simulink model "Learning_Example_run"  (R2020b)
settings: Solver=VariableStepAuto  StartTime=0.0  StopTime=50  RelTol=1e-3
values from neighbouring files (symbols this model uses):
  delta_time = 0.0178961433409    [Angular_gust.mat]    (also in Linear_gust.mat; Real_Values.m = time/length(xdata); Trial_Script.m = time/length(xdata); TryingNewAeroCoeffs.m = time/length(xdata))
  Fb1_l = -2600    [Angular_gust.mat]    (also in Linear_gust.mat; Real_Values.m = -260; Trial_Script.m; TryingNewAeroCoeffs.m)
  Fb1_u = 2600    [Angular_gust.mat]    (also in Linear_gust.mat; Real_Values.m = 260; Trial_Script.m; TryingNewAeroCoeffs.m)
  Fb2_l = -2600    [Angular_gust.mat]    (also in Linear_gust.mat; Real_Values.m = -260; Trial_Script.m; TryingNewAeroCoeffs.m)
  Fb2_u = 2600    [Angular_gust.mat]    (also in Linear_gust.mat; Real_Values.m = 260; Trial_Script.m; TryingNewAeroCoeffs.m)
  Fb3_l = -3200    [Angular_gust.mat]    (also in Linear_gust.mat; Real_Values.m = -320; Trial_Script.m; TryingNewAeroCoeffs.m)
  Fb3_u = 3200    [Angular_gust.mat]    (also in Linear_gust.mat; Real_Values.m = 320; Trial_Script.m; TryingNewAeroCoeffs.m)
  Fb4_l = -3200    [Angular_gust.mat]    (also in Linear_gust.mat; Real_Values.m = -320; Trial_Script.m; TryingNewAeroCoeffs.m)
  Fb4_u = 3200    [Angular_gust.mat]    (also in Linear_gust.mat; Real_Values.m = 320; Trial_Script.m; TryingNewAeroCoeffs.m)
  Fc1_l = -300    [Angular_gust.mat]    (also in Linear_gust.mat; Real_Values.m = -100; Trial_Script.m = -3000; TryingNewAeroCoeffs.m)
  Fc1_u = 300    [Angular_gust.mat]    (also in Linear_gust.mat; Real_Values.m = 100; Trial_Script.m = 3000; TryingNewAeroCoeffs.m)
  Fc2_l = -300    [Angular_gust.mat]    (also in Linear_gust.mat; Real_Values.m = -100; Trial_Script.m = -3000; TryingNewAeroCoeffs.m)
  Fc2_u = 300    [Angular_gust.mat]    (also in Linear_gust.mat; Real_Values.m = 100; Trial_Script.m = 3000; TryingNewAeroCoeffs.m)
  Fc3_l = -300    [Angular_gust.mat]    (also in Linear_gust.mat; Real_Values.m = -100; Trial_Script.m = -3000; TryingNewAeroCoeffs.m)
  Fc3_u = 300    [Angular_gust.mat]    (also in Linear_gust.mat; Real_Values.m = 100; Trial_Script.m = 3000; TryingNewAeroCoeffs.m)
  fprop = 1000    [Angular_gust.mat]    (also in Linear_gust.mat; TryingNewAeroCoeffs.m)
  Ft1_l = -5600    [Angular_gust.mat]    (also in Linear_gust.mat; Real_Values.m = -560; Trial_Script.m; TryingNewAeroCoeffs.m)
  Ft1_u = 5600    [Angular_gust.mat]    (also in Linear_gust.mat; Real_Values.m = 560; Trial_Script.m; TryingNewAeroCoeffs.m)
  Ft2_l = -5600    [Angular_gust.mat]    (also in Linear_gust.mat; Real_Values.m = -560; Trial_Script.m; TryingNewAeroCoeffs.m)
  Ft2_u = 5600    [Angular_gust.mat]    (also in Linear_gust.mat; Real_Values.m = 560; Trial_Script.m; TryingNewAeroCoeffs.m)
  Ft3_l = -3200    [Angular_gust.mat]    (also in Linear_gust.mat; Real_Values.m = -320; Trial_Script.m; TryingNewAeroCoeffs.m)
  Ft3_u = 3200    [Angular_gust.mat]    (also in Linear_gust.mat; Real_Values.m = 320; Trial_Script.m; TryingNewAeroCoeffs.m)
  Ft4_l = -3200    [Angular_gust.mat]    (also in Linear_gust.mat; Real_Values.m = -320; Trial_Script.m; TryingNewAeroCoeffs.m)
  Ft4_u = 3200    [Angular_gust.mat]    (also in Linear_gust.mat; Real_Values.m = 320; Trial_Script.m; TryingNewAeroCoeffs.m)
  g = 9.81    [Angular_gust.mat]    (also in Linear_gust.mat; Real_Values.m; Trial_Script.m; TryingNewAeroCoeffs.m)
  m = 941.102    [Angular_gust.mat]    (also in Linear_gust.mat; Real_Values.m; Trial_Script.m = 645; TryingNewAeroCoeffs.m)
  r_cgCatia = [0.0401998 0.00180957 -0.293434]    [Angular_gust.mat]    (also in Linear_gust.mat; Real_Values.m = TcgCatia*r_cgCatia; Trial_Script.m = [2; 0; 0]; TryingNewAeroCoeffs.m = TcgCatia*r_cgCatia)
  r_trajectory = [0 0 0]    [Angular_gust.mat]    (also in Linear_gust.mat; Real_Values.m = [0;0;0]; Trial_Script.m = [0;0;0]; TryingNewAeroCoeffs.m = [0;0;0])
  rho = 1.225    [Angular_gust.mat]    (also in Linear_gust.mat; Real_Values.m; Trial_Script.m; TryingNewAeroCoeffs.m)
  t_finalgust = 17.9140394843    [Angular_gust.mat]    (also in Linear_gust.mat; Real_Values.m = time; TryingNewAeroCoeffs.m = time)
  TcgCatia = [1  0  0; 0  -1  0; 0  0  -1]    [Angular_gust.mat]    (also in Linear_gust.mat; Real_Values.m = [1 0 0; Trial_Script.m = [1 0 0; TryingNewAeroCoeffs.m = [1 0 0)
  time = 17.9140394843    [Angular_gust.mat]    (also in Linear_gust.mat; Real_Values.m = rdiff_abs/V0_shard; Trial_Script.m = abs(rdiff_shard(2)/V0_shard(2)); TryingNewAeroCoeffs.m = rdiff_abs/V0_shard)
  time_delay = 0.01    [Angular_gust.mat]    (also in Linear_gust.mat; Real_Values.m = 0.1; Trial_Script.m = 0.1; TryingNewAeroCoeffs.m)
  Tzy_Shard = [6.12323399574e-17  1  1.22464679915e-16; 1  -6.12323399574e-17  -7.49879891331e-33; 0  1.22464679915e-16  -1]    [Angular_gust.mat]    (also in Linear_gust.mat; Real_Values.m = [cos(pi/2) -sin(pi/2) 0; sin(pi/2) cos(pi/2) 0; 0 0 1]*[1 0 ; Trial_Script.m = [cos(pi/2) -sin(pi/2) 0; sin(pi/2) cos(pi/2) 0; 0 0 1]*[1 0 ; TryingNewAeroCoeffs.m = [cos(pi/2) -sin(pi/2) 0; sin(pi/2) cos(pi/2) 0; 0 0 1]*[1 0 )
  u0_final = 23.9559    [Angular_gust.mat]    (also in Linear_gust.mat; Real_Values.m = u_0(length(u_0)); TryingNewAeroCoeffs.m = u_0(length(u_0)))
  u0_ini = 24.7775    [Angular_gust.mat]    (also in Linear_gust.mat; TryingNewAeroCoeffs.m = u_0(1))
  u1_final = -0.480858    [Angular_gust.mat]    (also in Linear_gust.mat; Real_Values.m = u_1(length(u_1)); TryingNewAeroCoeffs.m = u_1(length(u_1)))
  u1_ini = 0.712897    [Angular_gust.mat]    (also in Linear_gust.mat; TryingNewAeroCoeffs.m = u_1(1))
  u2_final = -0.725589    [Angular_gust.mat]    (also in Linear_gust.mat; Real_Values.m = u_2(length(u_2)); TryingNewAeroCoeffs.m = u_2(length(u_2)))
  u2_ini = -0.504815    [Angular_gust.mat]    (also in Linear_gust.mat; TryingNewAeroCoeffs.m = u_2(1))
  u_0 = [24.7775 24.7775 24.7775 24.7775 24.7775 24.7775 24.7775 24.7775 24.7775 24.7775 24.7775 24.7775 ... (1001 elements, 1001x1)]    [Angular_gust.mat]    (also in Linear_gust.mat; Real_Values.m = a(1:d_shard,1); Trial_Script.m = a(1:d_shard,1); TryingNewAeroCoeffs.m = a(1:d_shard,1))
  u_1 = [0.712897 0.712897 0.712897 0.712897 0.712897 0.712897 0.712897 0.712897 0.712897 0.712897 0.712897 0.712897 ... (1001 elements, 1001x1)]    [Angular_gust.mat]    (also in Linear_gust.mat; Real_Values.m = a(1:d_shard,2); Trial_Script.m = a(1:d_shard,2); TryingNewAeroCoeffs.m = a(1:d_shard,2))
  u_2 = [-0.504815 -0.504815 -0.504815 -0.504815 -0.504815 -0.504815 -0.504815 -0.504815 -0.504815 -0.504815 -0.504815 -0.504815 ... (1001 elements, 1001x1)]    [Angular_gust.mat]    (also in Linear_gust.mat; Real_Values.m = a(1:d_shard,3); Trial_Script.m = a(1:d_shard,3); TryingNewAeroCoeffs.m = a(1:d_shard,3))
  v_sh = [9.97862823256 -6.11014756245e-16 -13.3493354282]    [Angular_gust.mat]    (also in Linear_gust.mat; TryingNewAeroCoeffs.m = Tzy_Shard*[0; Vz0_shard; Vy0_shard])
  vq1 = interp1(out.tout,Fx_pre,xq)    [Learning_Code.m]    (also in PlottingSigmoidLeftover.m)
  vq2 = interp1(out.tout,Fy_pre,xq)    [Learning_Code.m]    (also in PlottingSigmoidLeftover.m)
  vq3 = interp1(out.tout,Fz_pre,xq)    [Learning_Code.m]    (also in PlottingSigmoidLeftover.m)
  xq = 0:0.001:40    [Learning_Code.m]    (also in PlottingSigmoidLeftover.m)
  ZI_Cx = [4.10002314469 4.10486511138 4.10970707807 4.11454904475 4.11939101144 4.12423297813 4.12907494481 4.1339169115 4.13875887819 4.14360084487 4.14844281156 4.15328477825 ... (65341 elements, 361x181)]    [Angular_gust.mat]    (also in Linear_gust.mat; Real_Values.m = model_Cx(XI_Cx, YI_Cx); Trial_Script.m = model_Cx(XI_Cx, YI_Cx); TryingNewAeroCoeffs.m = model_Cx(XI_Cx, YI_Cx))
  ZI_Cy = [5.10662222372 5.15407485934 5.20152749496 5.24898013059 5.29643276621 5.34388540184 5.39133803746 5.43879067308 5.48624330871 5.53369594433 5.58114857996 5.62860121558 ... (65341 elements, 361x181)]    [Angular_gust.mat]    (also in Linear_gust.mat; Real_Values.m = model_Cy(XI_Cy, YI_Cy); Trial_Script.m = model_Cy(XI_Cy, YI_Cy); TryingNewAeroCoeffs.m = model_Cy(XI_Cy, YI_Cy))
  ZI_Cz = [-10.5947720774 -10.6317912004 -10.6688103235 -10.7058294465 -10.7428485695 -10.7798676926 -10.8168868156 -10.8539059387 -10.8909250617 -10.9279441847 -10.9649633078 -11.0019824308 ... (65341 elements, 361x181)]    [Angular_gust.mat]    (also in Linear_gust.mat; Real_Values.m = model_Cz(XI_Cz, YI_Cz); Trial_Script.m = model_Cz(XI_Cz, YI_Cz); TryingNewAeroCoeffs.m = model_Cz(XI_Cz, YI_Cz))
  ZI_p = [6.05111971338 6.06712776392 6.08313581446 6.099143865 6.11515191553 6.13115996607 6.14716801661 6.16317606715 6.17918411769 6.19519216823 6.21120021877 6.22720826931 ... (65341 elements, 361x181)]    [Angular_gust.mat]    (also in Linear_gust.mat; Real_Values.m = model_p(XI_p, YI_p); Trial_Script.m = model_p(XI_p, YI_p); TryingNewAeroCoeffs.m = model_p(XI_p, YI_p))
  ZI_q = [0.071083987219 0.054175962948 0.0372679386771 0.0203599144061 0.00345189013513 -0.0134561341358 -0.0303641584068 -0.0472721826778 -0.0641802069487 -0.0810882312197 -0.0979962554907 -0.114904279762 ... (65341 elements, 361x181)]    [Angular_gust.mat]    (also in Linear_gust.mat; Real_Values.m = model_q(XI_q, YI_q); Trial_Script.m = model_q(XI_q, YI_q); TryingNewAeroCoeffs.m = model_q(XI_q, YI_q))
  ZI_r = [-1.8762921931 -1.88364224017 -1.89099228723 -1.8983423343 -1.90569238136 -1.91304242842 -1.92039247549 -1.92774252255 -1.93509256961 -1.94244261668 -1.94979266374 -1.95714271081 ... (65341 elements, 361x181)]    [Angular_gust.mat]    (also in Linear_gust.mat; Real_Values.m = model_r(XI_r, YI_r); Trial_Script.m = model_r(XI_r, YI_r); TryingNewAeroCoeffs.m = model_r(XI_r, YI_r))
libraries: dspsigops x11, simulink x6, pid_lib x3, sharedutil x1
settings Model: Creator=Jonathan van Zyl  LastModifiedBy=Jonathan van Zyl

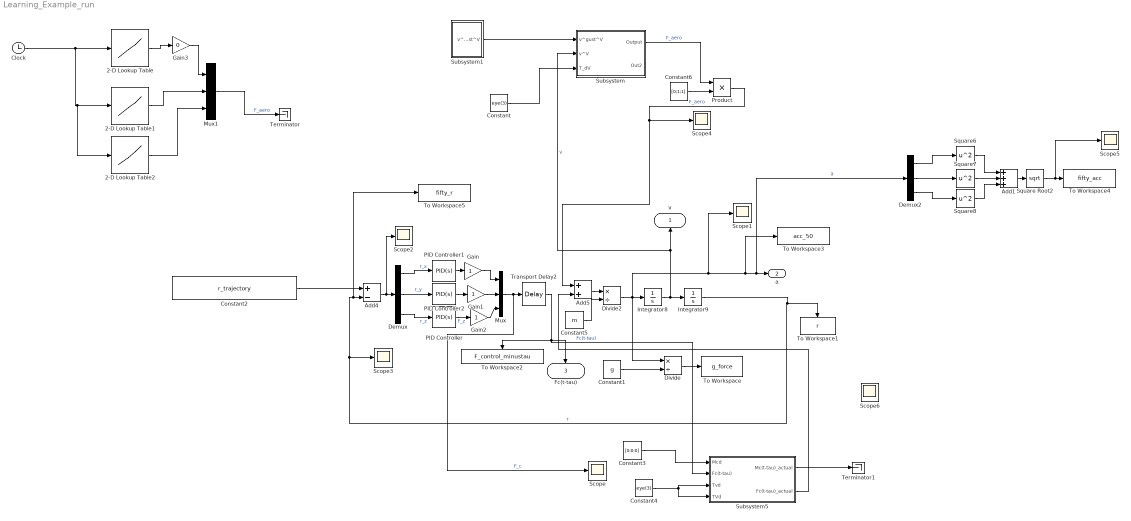
== system Learning_Example_run ==
  2-D Lookup Table : Lookup_n-D  NumberOfTableDimensions=1  BreakpointsForDimension1=xq  BreakpointsForDimension2=[0:1:40001]  Table=vq1  InternalRulePriority=Speed  RndMeth=Simplest  InputSameDT=on
  2-D Lookup Table1 : Lookup_n-D  NumberOfTableDimensions=1  BreakpointsForDimension1=xq  BreakpointsForDimension2=[0:1:40001]  Table=vq2  InternalRulePriority=Speed  RndMeth=Simplest  InputSameDT=on
  2-D Lookup Table2 : Lookup_n-D  NumberOfTableDimensions=1  BreakpointsForDimension1=xq  BreakpointsForDimension2=[0:1:40001]  Table=vq3  InternalRulePriority=Speed  RndMeth=Simplest  InputSameDT=on
  Add1 : Sum  Inputs=+++
  Add4 : Sum  Inputs=+-
  Add5 : Sum
  Clock : Clock
  Constant : Constant  Value=eye(3)
  Constant1 : Constant  Value=g
  Constant2 : Constant  Value=r_trajectory
  Constant3 : Constant  Value=[0;0;0]
  Constant4 : Constant  Value=eye(3)
  Constant5 : Constant  Value=m
  Constant6 : Constant  Value=[0;1;1]
  Demux : Demux  Outputs=3
  Demux2 : Demux  Outputs=3
  Divide : Product  Inputs=*/
  Divide2 : Product  Inputs=*/
  Gain : Gain
  Gain1 : Gain
  Gain2 : Gain
  Gain3 : Gain  Gain=0
  Integrator8 : Integrator
  Integrator9 : Integrator
  Mux : Mux  Inputs=3
  Mux1 : Mux  Inputs=3
  PID Controller : pid_lib/PID Controller  Controller=PID  Form=Parallel  TimeDomain=Continuous-time  UseExternalTs=off  SampleTime=-1  IntegratorMethod=Forward Euler  FilterMethod=Forward Euler  ControllerParametersSource=internal  P=165.49617069696  I=7.27585376172433  D=919.065111272192  UseFilter=on  N=5.45397025421619  TunerSelectOption=Transfer Function Based (PID Tuner App)  InitialConditionSource=internal  InitialConditionForIntegrator=0  InitialConditionForFilter=0  DifferentiatorICPrevScaledInput=0  ExternalReset=none  TrackingMode=off  Kt=1  LimitOutput=off  SatLimitsSource=internal  UpperSaturationLimit=inf  LowerSaturationLimit=-inf  LinearizeAsGain=on  AntiWindupMode=none  Kb=1  POutMin=[]  POutMax=[]  IOutMin=[]  IOutMax=[]  DOutMin=[]  DOutMax=[]  NOutMin=[]  NOutMax=[]  SumOutMin=[]  SumOutMax=[]  SaturationOutMin=[]  SaturationOutMax=[]  PParamMin=[]  PParamMax=[]  IParamMin=[]  IParamMax=[]  DParamMin=[]  DParamMax=[]  NParamMin=[]  NParamMax=[]  KbParamMin=[]  KbParamMax=[]  KtParamMin=[]  KtParamMax=[]  KbOutMin=[]  KbOutMax=[]  KtOutMin=[]  KtOutMax=[]  IntegratorOutMin=[]  IntegratorOutMax=[]  FilterOutMin=[]  FilterOutMax=[]  SumI1OutMin=[]  SumI1OutMax=[]  SumI2OutMin=[]  SumI2OutMax=[]  SumI3OutMin=[]  SumI3OutMax=[]  SumI4OutMin=[]  SumI4OutMax=[]  SumDOutMin=[]  SumDOutMax=[]  DifferentiatorOutMin=[]  DifferentiatorOutMax=[]  FilterDiffOutCoefMin=[]  FilterDiffOutCoefMax=[]  ReciprocalOutMin=[]  ReciprocalOutMax=[]  SumDenOutMin=[]  SumDenOutMax=[]  SumNumOutMin=[]  SumNumOutMax=[]  DivideOutMin=[]  DivideOutMax=[]  UdiffTsProdOutMin=[]  UdiffTsProdOutMax=[]  NTsProdOutMin=[]  NTsProdOutMax=[]  UintegralTsProdOutMin=[]  UintegralTsProdOutMax=[]  UngainTsProdOutMin=[]  UngainTsProdOutMax=[]  IntegratorContinuousStateAttributes=''  IntegratorStateMustResolveToSignalObject=off  IntegratorRTWStateStorageClass=Auto  FilterContinuousStateAttributes=''  FilterStateMustResolveToSignalObject=off  FilterRTWStateStorageClass=Auto  ParallelPVariant=InternalParameters  IdealPVariant=Disabled  IVariant=InternalParameters  DVariant=InternalParameters  IntegratorVariant=Continuous  SatVariant=Disabled  AWVariant=Passthrough  PCopyVariant=Disabled  TRVariant=Disabled  FdbkBlocksVariant=Forward  IdealPFdbkVariant=Disabled  SatFdbkVariant=Disabled  DerivativeFilterVariant=ContFilter  NVariant=InternalParameters  NCopyVariant=Disabled  FilterICVariant=InternalICsFilter  IntegratorICVariant=InternalICs  ExternalResetVariant=Disabled  TRSumVariant=Passthrough  SumFdbkVariant=Disabled  SumVariant=Sum_PID  TsampFilterVariant=InternalTs  TsampNgainVariant=Passthrough  TsampIntegralVariant=Passthrough  ExternalSaturationOutDataTypeStr=Inherit: Same as second input
  PID Controller1 : pid_lib/PID Controller  Controller=PID  Form=Parallel  TimeDomain=Continuous-time  UseExternalTs=off  SampleTime=-1  IntegratorMethod=Forward Euler  FilterMethod=Forward Euler  ControllerParametersSource=internal  P=118.225343121314  I=1.50893910785693  D=2058.11872086996  UseFilter=on  N=250.023518875976  TunerSelectOption=Transfer Function Based (PID Tuner App)  InitialConditionSource=internal  InitialConditionForIntegrator=0  InitialConditionForFilter=0  DifferentiatorICPrevScaledInput=0  ExternalReset=none  TrackingMode=off  Kt=1  LimitOutput=off  SatLimitsSource=internal  UpperSaturationLimit=inf  LowerSaturationLimit=-inf  LinearizeAsGain=on  AntiWindupMode=none  Kb=1  POutMin=[]  POutMax=[]  IOutMin=[]  IOutMax=[]  DOutMin=[]  DOutMax=[]  NOutMin=[]  NOutMax=[]  SumOutMin=[]  SumOutMax=[]  SaturationOutMin=[]  SaturationOutMax=[]  PParamMin=[]  PParamMax=[]  IParamMin=[]  IParamMax=[]  DParamMin=[]  DParamMax=[]  NParamMin=[]  NParamMax=[]  KbParamMin=[]  KbParamMax=[]  KtParamMin=[]  KtParamMax=[]  KbOutMin=[]  KbOutMax=[]  KtOutMin=[]  KtOutMax=[]  IntegratorOutMin=[]  IntegratorOutMax=[]  FilterOutMin=[]  FilterOutMax=[]  SumI1OutMin=[]  SumI1OutMax=[]  SumI2OutMin=[]  SumI2OutMax=[]  SumI3OutMin=[]  SumI3OutMax=[]  SumI4OutMin=[]  SumI4OutMax=[]  SumDOutMin=[]  SumDOutMax=[]  DifferentiatorOutMin=[]  DifferentiatorOutMax=[]  FilterDiffOutCoefMin=[]  FilterDiffOutCoefMax=[]  ReciprocalOutMin=[]  ReciprocalOutMax=[]  SumDenOutMin=[]  SumDenOutMax=[]  SumNumOutMin=[]  SumNumOutMax=[]  DivideOutMin=[]  DivideOutMax=[]  UdiffTsProdOutMin=[]  UdiffTsProdOutMax=[]  NTsProdOutMin=[]  NTsProdOutMax=[]  UintegralTsProdOutMin=[]  UintegralTsProdOutMax=[]  UngainTsProdOutMin=[]  UngainTsProdOutMax=[]  IntegratorContinuousStateAttributes=''  IntegratorStateMustResolveToSignalObject=off  IntegratorRTWStateStorageClass=Auto  FilterContinuousStateAttributes=''  FilterStateMustResolveToSignalObject=off  FilterRTWStateStorageClass=Auto  ParallelPVariant=InternalParameters  IdealPVariant=Disabled  IVariant=InternalParameters  DVariant=InternalParameters  IntegratorVariant=Continuous  SatVariant=Disabled  AWVariant=Passthrough  PCopyVariant=Disabled  TRVariant=Disabled  FdbkBlocksVariant=Forward  IdealPFdbkVariant=Disabled  SatFdbkVariant=Disabled  DerivativeFilterVariant=ContFilter  NVariant=InternalParameters  NCopyVariant=Disabled  FilterICVariant=InternalICsFilter  IntegratorICVariant=InternalICs  ExternalResetVariant=Disabled  TRSumVariant=Passthrough  SumFdbkVariant=Disabled  SumVariant=Sum_PID  TsampFilterVariant=InternalTs  TsampNgainVariant=Passthrough  TsampIntegralVariant=Passthrough  ExternalSaturationOutDataTypeStr=Inherit: Same as second input
  PID Controller2 : pid_lib/PID Controller  Controller=PID  Form=Parallel  TimeDomain=Continuous-time  UseExternalTs=off  SampleTime=-1  IntegratorMethod=Forward Euler  FilterMethod=Forward Euler  ControllerParametersSource=internal  P=165.49617069696  I=7.27585376172433  D=919.065111272192  UseFilter=on  N=5.45397025421619  TunerSelectOption=Transfer Function Based (PID Tuner App)  InitialConditionSource=internal  InitialConditionForIntegrator=0  InitialConditionForFilter=0  DifferentiatorICPrevScaledInput=0  ExternalReset=none  TrackingMode=off  Kt=1  LimitOutput=off  SatLimitsSource=internal  UpperSaturationLimit=inf  LowerSaturationLimit=-inf  LinearizeAsGain=on  AntiWindupMode=none  Kb=1  POutMin=[]  POutMax=[]  IOutMin=[]  IOutMax=[]  DOutMin=[]  DOutMax=[]  NOutMin=[]  NOutMax=[]  SumOutMin=[]  SumOutMax=[]  SaturationOutMin=[]  SaturationOutMax=[]  PParamMin=[]  PParamMax=[]  IParamMin=[]  IParamMax=[]  DParamMin=[]  DParamMax=[]  NParamMin=[]  NParamMax=[]  KbParamMin=[]  KbParamMax=[]  KtParamMin=[]  KtParamMax=[]  KbOutMin=[]  KbOutMax=[]  KtOutMin=[]  KtOutMax=[]  IntegratorOutMin=[]  IntegratorOutMax=[]  FilterOutMin=[]  FilterOutMax=[]  SumI1OutMin=[]  SumI1OutMax=[]  SumI2OutMin=[]  SumI2OutMax=[]  SumI3OutMin=[]  SumI3OutMax=[]  SumI4OutMin=[]  SumI4OutMax=[]  SumDOutMin=[]  SumDOutMax=[]  DifferentiatorOutMin=[]  DifferentiatorOutMax=[]  FilterDiffOutCoefMin=[]  FilterDiffOutCoefMax=[]  ReciprocalOutMin=[]  ReciprocalOutMax=[]  SumDenOutMin=[]  SumDenOutMax=[]  SumNumOutMin=[]  SumNumOutMax=[]  DivideOutMin=[]  DivideOutMax=[]  UdiffTsProdOutMin=[]  UdiffTsProdOutMax=[]  NTsProdOutMin=[]  NTsProdOutMax=[]  UintegralTsProdOutMin=[]  UintegralTsProdOutMax=[]  UngainTsProdOutMin=[]  UngainTsProdOutMax=[]  IntegratorContinuousStateAttributes=''  IntegratorStateMustResolveToSignalObject=off  IntegratorRTWStateStorageClass=Auto  FilterContinuousStateAttributes=''  FilterStateMustResolveToSignalObject=off  FilterRTWStateStorageClass=Auto  ParallelPVariant=InternalParameters  IdealPVariant=Disabled  IVariant=InternalParameters  DVariant=InternalParameters  IntegratorVariant=Continuous  SatVariant=Disabled  AWVariant=Passthrough  PCopyVariant=Disabled  TRVariant=Disabled  FdbkBlocksVariant=Forward  IdealPFdbkVariant=Disabled  SatFdbkVariant=Disabled  DerivativeFilterVariant=ContFilter  NVariant=InternalParameters  NCopyVariant=Disabled  FilterICVariant=InternalICsFilter  IntegratorICVariant=InternalICs  ExternalResetVariant=Disabled  TRSumVariant=Passthrough  SumFdbkVariant=Disabled  SumVariant=Sum_PID  TsampFilterVariant=InternalTs  TsampNgainVariant=Passthrough  TsampIntegralVariant=Passthrough  ExternalSaturationOutDataTypeStr=Inherit: Same as second input
  Product : Product
  Scope{,1..6} (7 alike) : Scope
  Square Root2 : Sqrt  SaturateOnIntegerOverflow=on
  Square6 : Math  Operator=square  SaturateOnIntegerOverflow=on
  Square7 : Math  Operator=square  SaturateOnIntegerOverflow=on
  Square8 : Math  Operator=square  SaturateOnIntegerOverflow=on
  Subsystem : Subsystem
  Subsystem1 : Subsystem
  Subsystem5 : Subsystem
  Terminator : Terminator
  Terminator1 : Terminator
  To Workspace : ToWorkspace  VariableName=g_force  SaveFormat=Timeseries  SampleTime=-1
      settings: Save2DSignal=2-D array (concatenate along first dimension)
  To Workspace1 : ToWorkspace  VariableName=r  SaveFormat=Timeseries  SampleTime=-1
  To Workspace2 : ToWorkspace  VariableName=F_control_minustau  SaveFormat=Timeseries  SampleTime=-1
  To Workspace3 : ToWorkspace  VariableName=acc_50  SaveFormat=Timeseries  SampleTime=-1
  To Workspace4 : ToWorkspace  VariableName=fifty_acc  SaveFormat=Timeseries  SampleTime=-1
  To Workspace5 : ToWorkspace  VariableName=fifty_r  SaveFormat=Timeseries  SampleTime=-1
  Transport Delay2 : TransportDelay  DelayTime=time_delay  TransDelayFeedthrough=on
  v : Outport
  a : Outport  Port=2
  Fc(t-tau) : Outport  Port=3
  wires:
  Constant1/1 -> Divide/2
  Mux/1 -> Scope/1, Transport Delay2/1  "F_c"
  Demux/2 -> PID Controller2/1  "r_y"
  Divide2/1 -> Scope1/1, To Workspace3/1, Demux2/1, a/1, Integrator8/1, Divide/1  "a"
  Gain/1 -> Mux/1
  Gain1/1 -> Mux/2
  Add4/1 -> Scope2/1, Demux/1
  Integrator9/1 -> Scope3/1, To Workspace5/1, Add4/2, To Workspace1/1  "r"
  Gain2/1 -> Mux/3
  Demux/3 -> PID Controller/1  "r_z"
  Constant2/1 -> Add4/1
  Constant5/1 -> Divide2/2
  PID Controller1/1 -> Gain/1
  PID Controller2/1 -> Gain1/1
  Product/1 -> Scope4/1, Add5/1  "F_aero"
  Divide/1 -> To Workspace/1
  Add5/1 -> Divide2/1
  PID Controller/1 -> Gain2/1  "F_z"
  Transport Delay2/1 -> Subsystem5/2(Fc(t-tau)), Fc(t-tau)/1, To Workspace2/1  "Fc(t-tau)"
  Demux/1 -> PID Controller1/1  "r_x"
  Clock/1 -> 2-D Lookup Table2/1, 2-D Lookup Table1/1, 2-D Lookup Table/1
  2-D Lookup Table/1 -> Gain3/1
  Gain3/1 -> Mux1/1
  2-D Lookup Table1/1 -> Mux1/2
  2-D Lookup Table2/1 -> Mux1/3
  Constant/1 -> Subsystem/3(T_dV)
  Subsystem1/1(v^gust^V) -> Subsystem/1(v^gust^V)
  Integrator8/1 -> Subsystem/2(v^V), v/1, Integrator9/1  "v"
  Mux1/1 -> Terminator/1  "F_aero"
  Constant3/1 -> Subsystem5/1(Mcd)
  Constant4/1 -> Subsystem5/3(Tvd), Subsystem5/4(TVd)
  Subsystem5/2(Fc(t-tau)_actual) -> Add5/2
  Subsystem5/1(Mc(t-tau)_actual) -> Terminator1/1
  Constant6/1 -> Product/2
  Subsystem/1(Output) -> Product/1  "F_aero"
  Demux2/3 -> Square8/1
  Demux2/2 -> Square7/1
  Square8/1 -> Add1/3
  Demux2/1 -> Square6/1
  Square7/1 -> Add1/2
  Add1/1 -> Square Root2/1
  Square6/1 -> Add1/1
  Square Root2/1 -> Scope5/1, To Workspace4/1

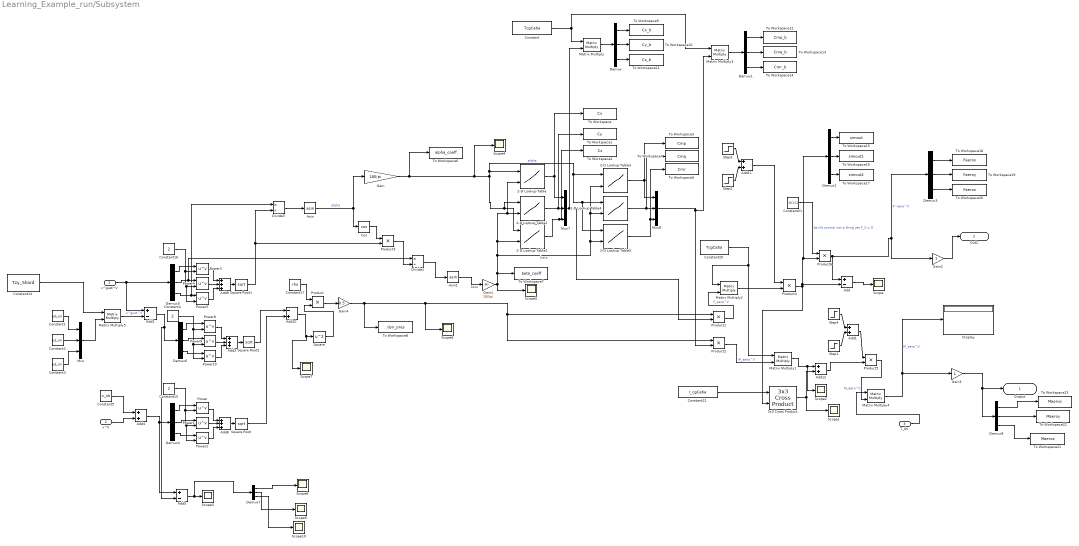
== system Learning_Example_run/Subsystem ==
  v^gust^V : Inport
  v^V : Inport  Port=2
  T_dV : Inport  Port=3
  2-D Lookup Table : Lookup_n-D  BreakpointsForDimension1=[-180:1:180]  BreakpointsForDimension2=[-90:1:90]  Table=ZI_Cx  InternalRulePriority=Speed  RndMeth=Simplest  InputSameDT=on
      settings: InputPortMap=u0,u1
  2-D Lookup Table1 : Lookup_n-D  BreakpointsForDimension1=[-180:1:180]  BreakpointsForDimension2=[-90:1:90]  Table=ZI_Cy  InternalRulePriority=Speed  RndMeth=Simplest  InputSameDT=on
      settings: InputPortMap=u0,u1
  2-D Lookup Table2 : Lookup_n-D  BreakpointsForDimension1=[-180:1:180]  BreakpointsForDimension2=[-90:1:90]  Table=ZI_Cz  InternalRulePriority=Speed  RndMeth=Simplest  InputSameDT=on
      settings: InputPortMap=u0,u1
  2-D Lookup Table3 : Lookup_n-D  BreakpointsForDimension1=[-180:1:180]  BreakpointsForDimension2=[-90:1:90]  Table=ZI_p  InternalRulePriority=Speed  RndMeth=Simplest  InputSameDT=on
      settings: InputPortMap=u0,u1
  2-D Lookup Table4 : Lookup_n-D  BreakpointsForDimension1=[-180:1:180]  BreakpointsForDimension2=[-90:1:90]  Table=ZI_q  InternalRulePriority=Speed  RndMeth=Simplest  InputSameDT=on
      settings: InputPortMap=u0,u1
  2-D Lookup Table5 : Lookup_n-D  BreakpointsForDimension1=[-180:1:180]  BreakpointsForDimension2=[-90:1:90]  Table=ZI_r  InternalRulePriority=Speed  RndMeth=Simplest  InputSameDT=on
      settings: InputPortMap=u0,u1
  3x3 Cross Product : sharedutil/3x3 Cross Product  aMode=aMode
      settings: SourceProductBaseCode=AE,PW,MT,UV,VE,VP
  Add : Sum  Inputs=+-
  Add{1,4,11..12} (4 alike) : Sum
  Add10 : Sum  Inputs=-+
  Add2 : Sum  Inputs=+-
  Add3 : Sum  Inputs=+++
  Add5 : Sum  Inputs=+-
  Add8 : Sum  Inputs=+++
  Add9 : Sum  Inputs=+++
  Asin : Trigonometry  Operator=asin
  Asin1 : Trigonometry  Operator=asin
  Constant : Constant  Value=TcgCatia
  Constant1 : Constant  Value=u0_ini
  Constant14 : Constant  Value=Tzy_Shard
  Constant15 : Constant  Value=2
  Constant16 : Constant  Value=2
  Constant17 : Constant  Value=rho
  Constant2 : Constant  Value=u1_ini
  Constant20 : Constant  Value=TcgCatia
  Constant21 : Constant  Value=[0;1;1]
  Constant22 : Constant  Value=r_cgCatia
  Constant3 : Constant  Value=u2_ini
  Constant4 : Constant  Value=2
  Constant5 : Constant  Value=v_sh
  Cos : Trigonometry  Operator=cos
  Demux{,1..8} (9 alike) : Demux  Outputs=3
  Display : Display
  Divide1 : Product  Inputs=*/
  Divide3 : Product  Inputs=*/
  Gain : Gain  Gain=180/pi
  Gain1 : Gain  Gain=180/pi
  Gain2 : Gain
  Gain3 : Gain
  Gain4 : Gain  Gain=0.5
  Matrix Multiply{,1..5} (6 alike) : Product  Multiplication=Matrix(*)
  Mux : Mux  Inputs=3
  Mux7 : Mux  Inputs=3
  Mux8 : Mux  Inputs=3
  Power{,1..5,8..10} (9 alike) : Math  Operator=pow  SaturateOnIntegerOverflow=on
  Product{,1..6} (7 alike) : Product
  Scope{,1..10} (11 alike) : Scope
  Square : Math  Operator=square  SaturateOnIntegerOverflow=on
  Square Root : Sqrt  SaturateOnIntegerOverflow=on
  Square Root1 : Sqrt  SaturateOnIntegerOverflow=on
  Square Root2 : Sqrt  SaturateOnIntegerOverflow=on
  Step1 : Step  Time=0  SampleTime=0
  Step2 : Step  Time=0  SampleTime=0
  Step3 : Step  Time=time  After=-1  SampleTime=0
  Step4 : Step  Time=time  After=-1  SampleTime=0
  To Workspace : ToWorkspace  VariableName=Cx  SaveFormat=Timeseries  SampleTime=-1
  To Workspace1 : ToWorkspace  VariableName=Cy  SaveFormat=Timeseries  SampleTime=-1
  To Workspace10 : ToWorkspace  VariableName=Cy_b  SaveFormat=Timeseries  SampleTime=-1
  To Workspace11 : ToWorkspace  VariableName=Cz_b  SaveFormat=Timeseries  SampleTime=-1
  To Workspace12 : ToWorkspace  VariableName=Cmp_b  SaveFormat=Timeseries  SampleTime=-1
  To Workspace13 : ToWorkspace  VariableName=Cmq_b  SaveFormat=Timeseries  SampleTime=-1
  To Workspace14 : ToWorkspace  VariableName=Cmr_b  SaveFormat=Timeseries  SampleTime=-1
  To Workspace15 : ToWorkspace  VariableName=simout  SaveFormat=Timeseries  SampleTime=-1
  To Workspace16 : ToWorkspace  VariableName=simout1  SaveFormat=Timeseries  SampleTime=-1
  To Workspace17 : ToWorkspace  VariableName=simout2  SaveFormat=Timeseries  SampleTime=-1
  To Workspace18 : ToWorkspace  VariableName=Faerox  SaveFormat=Timeseries  SampleTime=-1
  To Workspace19 : ToWorkspace  VariableName=Faeroy  SaveFormat=Timeseries  SampleTime=-1
  To Workspace2 : ToWorkspace  VariableName=Cz  SaveFormat=Timeseries  SampleTime=-1
  To Workspace20 : ToWorkspace  VariableName=Faeroz  SaveFormat=Timeseries  SampleTime=-1
  To Workspace21 : ToWorkspace  VariableName=Maeroz  SaveFormat=Timeseries  SampleTime=-1
  To Workspace22 : ToWorkspace  VariableName=Maeroy  SaveFormat=Timeseries  SampleTime=-1
  To Workspace23 : ToWorkspace  VariableName=Maerox  SaveFormat=Timeseries  SampleTime=-1
  To Workspace3 : ToWorkspace  VariableName=Cmp  SaveFormat=Timeseries  SampleTime=-1
  To Workspace4 : ToWorkspace  VariableName=Cmq  SaveFormat=Timeseries  SampleTime=-1
  To Workspace5 : ToWorkspace  VariableName=Cmr  SaveFormat=Timeseries  SampleTime=-1
  To Workspace6 : ToWorkspace  VariableName=alpha_coeff  SaveFormat=Timeseries  SampleTime=-1
  To Workspace7 : ToWorkspace  VariableName=beta_coeff  SaveFormat=Timeseries  SampleTime=-1
  To Workspace8 : ToWorkspace  VariableName=dyn_pres  SaveFormat=Timeseries  SampleTime=-1
  To Workspace9 : ToWorkspace  VariableName=Cx_b  SaveFormat=Timeseries  SampleTime=-1
  Output : Outport
  Out2 : Outport  Port=2
  wires:
  Demux5/1 -> Power3/1
  Constant21/1 -> Product6/1  "As tilt control not a thing yet F_X = 0"
  2-D Lookup Table3/1 -> To Workspace3/1, Mux8/1
  Constant17/1 -> Product/1
  Power5/1 -> Add9/3
  Product4/1 -> Demux2/1, Product6/2, Add/2, 3x3 Cross Product/2
  Gain1/1 -> 2-D Lookup Table/2, 2-D Lookup Table1/2, 2-D Lookup Table2/2, 2-D Lookup Table3/2, 2-D Lookup Table4/2, 2-D Lookup Table5/2, To Workspace7/1, Scope5/1  "beta"
  2-D Lookup Table2/1 -> To Workspace2/1, Mux7/3
  Power3/1 -> Add9/1
  Constant15/1 -> Power2/2, Power1/2, Power/2
  Square/1 -> Product/2
  Demux4/2 -> Power1/1
  Gain4/1 -> To Workspace8/1, Scope6/1, Product2/1, Product1/1
  Square Root1/1 -> Product3/2, Divide3/2
  Product1/1 -> Matrix Multiply2/2  "F_aero^V"
  2-D Lookup Table1/1 -> To Workspace1/1, Mux7/2
  Add8/1 -> Square Root/1
  Cos/1 -> Product3/1
  3x3 Cross Product/1 -> Add12/2, Scope1/1
  Power2/1 -> Add8/3
  Add9/1 -> Square Root1/1
  Divide3/1 -> Asin/1
  Mux7/1 -> Matrix Multiply/2, Product1/2
  Demux5/2 -> Divide1/1, Power4/1
  Product3/1 -> Divide1/2
  Constant22/1 -> 3x3 Cross Product/1
  Product2/1 -> Matrix Multiply1/2  "M_aero^V"
  Demux4/3 -> Power2/1
  Square Root/1 -> Add10/2
  Constant16/1 -> Power5/2, Power4/2, Power3/2
  2-D Lookup Table5/1 -> To Workspace5/1, Mux8/3
  v^gust^V/1 -> Add2/1, Demux5/1
  Divide1/1 -> Asin1/1
  Power1/1 -> Add8/2
  Constant20/1 -> Matrix Multiply1/1, Matrix Multiply2/1
  Power4/1 -> Add9/2
  Power/1 -> Add8/1
  2-D Lookup Table4/1 -> To Workspace4/1, Mux8/2
  Matrix Multiply1/1 -> Scope2/1, Add12/1
  Mux8/1 -> Matrix Multiply3/2, Product2/2
  Demux4/1 -> Power/1
  Product6/1 -> Add/1, Demux3/1, Gain2/1  "F^aero^V"
  Demux5/3 -> Divide3/1, Power5/1
  Product/1 -> Gain4/1
  Gain/1 -> To Workspace6/1, Scope4/1, 2-D Lookup Table/1, 2-D Lookup Table5/1, 2-D Lookup Table4/1, 2-D Lookup Table3/1, 2-D Lookup Table2/1, 2-D Lookup Table1/1  "alpha"
  2-D Lookup Table/1 -> Mux7/1, To Workspace/1
  Add10/1 -> Scope7/1, Square/1
  Matrix Multiply4/1 -> Gain3/1, Display/1  "M_aero^V"
  T_dV/1 -> Matrix Multiply4/1
  v^V/1 -> Add4/2
  Add/1 -> Scope/1
  Constant/1 -> Matrix Multiply3/1, Matrix Multiply/1
  Matrix Multiply/1 -> Demux/1
  Demux/1 -> To Workspace9/1
  Demux/2 -> To Workspace10/1
  Demux/3 -> To Workspace11/1
  Matrix Multiply3/1 -> Demux1/1
  Demux1/1 -> To Workspace12/1
  Demux1/2 -> To Workspace13/1
  Demux1/3 -> To Workspace14/1
  Demux2/1 -> To Workspace15/1
  Demux2/2 -> To Workspace16/1
  Demux2/3 -> To Workspace17/1
  Demux3/1 -> To Workspace18/1
  Demux3/2 -> To Workspace19/1
  Demux3/3 -> To Workspace20/1
  Step3/1 -> Add11/1
  Add11/1 -> Product4/1
  Step2/1 -> Add11/2
  Matrix Multiply2/1 -> Product4/2
  Add1/1 -> Product5/1
  Step1/1 -> Add1/2
  Step4/1 -> Add1/1
  Product5/1 -> Matrix Multiply4/2  "M_aero^V"
  Add12/1 -> Product5/2
  Mux/1 -> Matrix Multiply5/2
  Constant3/1 -> Mux/3
  Constant1/1 -> Mux/1
  Constant2/1 -> Mux/2
  Add2/1 -> Add5/2, Demux6/1
  Constant14/1 -> Matrix Multiply5/1
  Matrix Multiply5/1 -> Add2/2  "v^gust^V"
  Power10/1 -> Add3/3
  Demux6/3 -> Power10/1
  Add3/1 -> Square Root2/1
  Power9/1 -> Add3/2
  Power8/1 -> Add3/1
  Demux6/2 -> Power9/1
  Demux6/1 -> Power8/1
  Square Root2/1 -> Add10/1
  Constant4/1 -> Power8/2, Power9/2, Power10/2
  Asin1/1 -> Gain1/1  "beta"
  Asin/1 -> Cos/1, Gain/1  "alpha"
  Constant5/1 -> Add4/1
  Add4/1 -> Add5/1, Demux4/1
  Add5/1 -> Demux7/1, Scope3/1
  Demux7/1 -> Scope8/1
  Demux7/2 -> Scope9/1
  Demux7/3 -> Scope10/1
  Gain2/1 -> Out2/1
  Gain3/1 -> Demux8/1, Output/1
  Demux8/3 -> To Workspace21/1
  Demux8/2 -> To Workspace22/1
  Demux8/1 -> To Workspace23/1

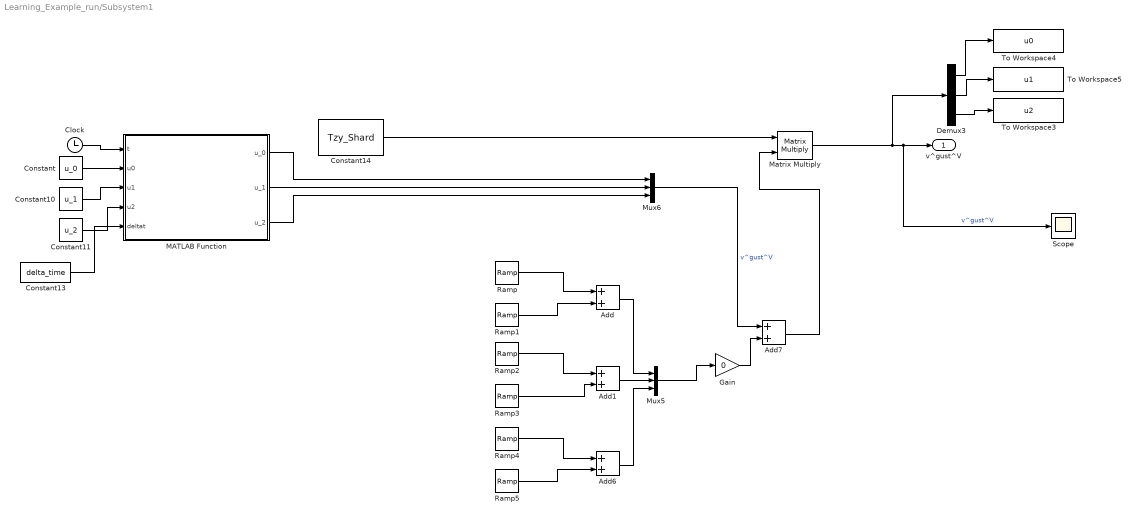
== system Learning_Example_run/Subsystem1 ==
  Add{,1,6..7} (4 alike) : Sum
  Clock : Clock
  Constant : Constant  Value=u_0
  Constant10 : Constant  Value=u_1
  Constant11 : Constant  Value=u_2
  Constant13 : Constant  Value=delta_time
  Constant14 : Constant  Value=Tzy_Shard
  Demux3 : Demux  Outputs=3
  Gain : Gain  Gain=0
  MATLAB Function : MATLAB Function  TreatAsAtomicUnit=on
  Matrix Multiply : Product  Multiplication=Matrix(*)
  Mux5 : Mux  Inputs=3
  Mux6 : Mux  Inputs=3
  Ramp : simulink/Sources/Ramp  slope=-1  start=t_finalgust  InitialOutput=0
  Ramp1 : simulink/Sources/Ramp  slope=1  start=t_finalgust + u0_final  InitialOutput=0
  Ramp2 : simulink/Sources/Ramp  slope=-1  start=t_finalgust  InitialOutput=0
  Ramp3 : simulink/Sources/Ramp  slope=1  start=t_finalgust + u1_final  InitialOutput=0
  Ramp4 : simulink/Sources/Ramp  slope=-1  start=t_finalgust  InitialOutput=0
  Ramp5 : simulink/Sources/Ramp  slope=1  start=t_finalgust + u2_final  InitialOutput=0
  Scope : Scope
  To Workspace3 : ToWorkspace  VariableName=u2  SaveFormat=Timeseries  SampleTime=-1
  To Workspace4 : ToWorkspace  VariableName=u0  SaveFormat=Timeseries  SampleTime=-1
  To Workspace5 : ToWorkspace  VariableName=u1  SaveFormat=Timeseries  SampleTime=-1
  v^gust^V : Outport
  wires:
  Add1/1 -> Mux5/2
  MATLAB Function/1(u_0) -> Mux6/1
  Add7/1 -> Matrix Multiply/2
  Constant13/1 -> MATLAB Function/5(deltat)
  Ramp4/1 -> Add6/1
  Ramp3/1 -> Add1/2
  Constant11/1 -> MATLAB Function/4(u2)
  Constant/1 -> MATLAB Function/2(u0)
  Ramp1/1 -> Add/2
  Mux5/1 -> Gain/1
  Constant14/1 -> Matrix Multiply/1
  MATLAB Function/2(u_1) -> Mux6/2
  Constant10/1 -> MATLAB Function/3(u1)
  Ramp/1 -> Add/1
  Matrix Multiply/1 -> Demux3/1, Scope/1, v^gust^V/1  "v^gust^V"
  Ramp5/1 -> Add6/2
  Add6/1 -> Mux5/3
  Clock/1 -> MATLAB Function/1(t)
  MATLAB Function/3(u_2) -> Mux6/3
  Add/1 -> Mux5/1
  Ramp2/1 -> Add1/1
  Mux6/1 -> Add7/1  "v^gust^V"
  Demux3/3 -> To Workspace3/1
  Demux3/2 -> To Workspace5/1
  Demux3/1 -> To Workspace4/1
  Gain/1 -> Add7/2

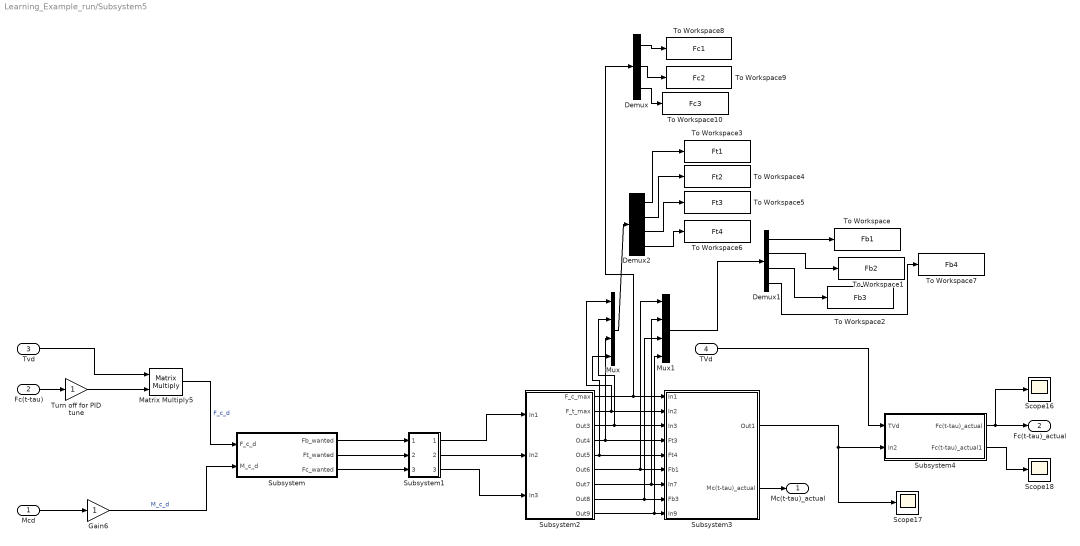
== system Learning_Example_run/Subsystem5 ==
  Mcd : Inport
  Fc(t-tau) : Inport  Port=2
  Tvd : Inport  Port=3
  TVd : Inport  Port=4
  Demux : Demux  Outputs=3
  Demux1 : Demux
  Demux2 : Demux
  Gain6 : Gain
  Matrix Multiply5 : Product  Multiplication=Matrix(*)
  Mux : Mux
  Mux1 : Mux
  Scope16 : Scope
  Scope17 : Scope
  Scope18 : Scope
  Subsystem : Subsystem
  Subsystem1 : Subsystem
  Subsystem2 : Subsystem
  Subsystem3 : Subsystem
  Subsystem4 : Subsystem
  To Workspace : ToWorkspace  VariableName=Fb1  SaveFormat=Timeseries  SampleTime=-1
  To Workspace1 : ToWorkspace  VariableName=Fb2  SaveFormat=Timeseries  SampleTime=-1
  To Workspace10 : ToWorkspace  VariableName=Fc3  SaveFormat=Timeseries  SampleTime=-1
  To Workspace2 : ToWorkspace  VariableName=Fb3  SaveFormat=Timeseries  SampleTime=-1
  To Workspace3 : ToWorkspace  VariableName=Ft1  SaveFormat=Timeseries  SampleTime=-1
  To Workspace4 : ToWorkspace  VariableName=Ft2  SaveFormat=Timeseries  SampleTime=-1
  To Workspace5 : ToWorkspace  VariableName=Ft3  SaveFormat=Timeseries  SampleTime=-1
  To Workspace6 : ToWorkspace  VariableName=Ft4  SaveFormat=Timeseries  SampleTime=-1
  To Workspace7 : ToWorkspace  VariableName=Fb4  SaveFormat=Timeseries  SampleTime=-1
  To Workspace8 : ToWorkspace  VariableName=Fc1  SaveFormat=Timeseries  SampleTime=-1
  To Workspace9 : ToWorkspace  VariableName=Fc2  SaveFormat=Timeseries  SampleTime=-1
  Turn off for PID tune : Gain
  Mc(t-tau)_actual : Outport
  Fc(t-tau)_actual : Outport  Port=2
  wires:
  Mcd/1 -> Gain6/1
  Turn off for PID tune/1 -> Matrix Multiply5/2
  Tvd/1 -> Matrix Multiply5/1
  Fc(t-tau)/1 -> Turn off for PID tune/1
  Matrix Multiply5/1 -> Subsystem/1(F_c_d)  "F_c_d"
  Gain6/1 -> Subsystem/2(M_c_d)  "M_c_d"
  Subsystem/1(Fb_wanted) -> Subsystem1/1(In1)
  Subsystem/2(Ft_wanted) -> Subsystem1/2(In2)
  Subsystem/3(Fc_wanted) -> Subsystem1/3(In3)
  Subsystem1/1(Out1) -> Subsystem2/1(In1)
  Subsystem1/2(Out2) -> Subsystem2/2(In2)
  Subsystem1/3(Out3) -> Subsystem2/3(In3)
  Subsystem3/1(Out1) -> Scope17/1, Subsystem4/2(In2)
  Subsystem2/1(F_c_max) -> Demux/1, Subsystem3/1(In1)
  Subsystem2/2(F_t_max) -> Mux/1, Subsystem3/2(In2)
  Subsystem2/3(Out3) -> Mux/2, Subsystem3/3(In3)
  Subsystem2/4(Out4) -> Subsystem3/4(Ft3), Mux/3
  Subsystem2/5(Out5) -> Subsystem3/5(Ft4), Mux/4
  Subsystem2/6(Out6) -> Mux1/1, Subsystem3/6(Fb1)
  Subsystem2/7(Out7) -> Mux1/2, Subsystem3/7(In7)
  Subsystem2/8(Out8) -> Subsystem3/8(Fb3), Mux1/3
  Subsystem2/9(Out9) -> Mux1/4, Subsystem3/9(In9)
  Subsystem3/2(Mc(t-tau)_actual) -> Mc(t-tau)_actual/1
  Subsystem4/1(Fc(t-tau)_actual) -> Scope16/1, Fc(t-tau)_actual/1
  TVd/1 -> Subsystem4/1(TVd)
  Subsystem4/2(Fc(t-tau)_actual1) -> Scope18/1
  Demux1/1 -> To Workspace/1
  Demux1/2 -> To Workspace1/1
  Demux1/3 -> To Workspace2/1
  Demux2/1 -> To Workspace3/1
  Demux2/2 -> To Workspace4/1
  Demux2/3 -> To Workspace5/1
  Demux2/4 -> To Workspace6/1
  Demux1/4 -> To Workspace7/1
  Demux/1 -> To Workspace8/1
  Demux/2 -> To Workspace9/1
  Demux/3 -> To Workspace10/1
  Mux/1 -> Demux2/1
  Mux1/1 -> Demux1/1

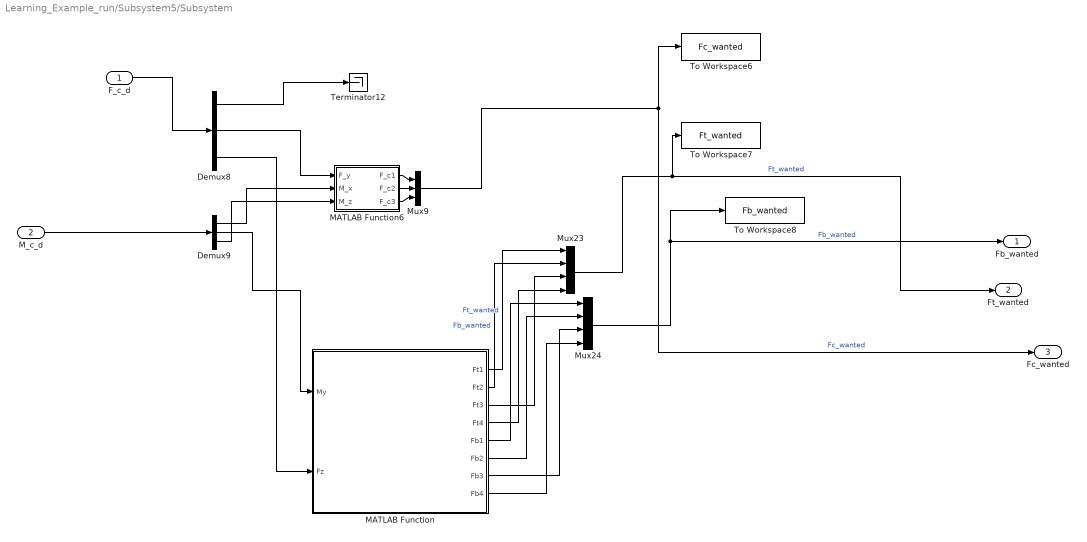
== system Learning_Example_run/Subsystem5/Subsystem ==
  F_c_d : Inport
  M_c_d : Inport  Port=2
  Demux8 : Demux  Outputs=3
  Demux9 : Demux  Outputs=3
  MATLAB Function : MATLAB Function  TreatAsAtomicUnit=on
  MATLAB Function6 : MATLAB Function  TreatAsAtomicUnit=on
  Mux23 : Mux
  Mux24 : Mux
  Mux9 : Mux  Inputs=3
  Terminator12 : Terminator
  To Workspace6 : ToWorkspace  VariableName=Fc_wanted  SaveFormat=Timeseries  SampleTime=-1
  To Workspace7 : ToWorkspace  VariableName=Ft_wanted  SaveFormat=Timeseries  SampleTime=-1
  To Workspace8 : ToWorkspace  VariableName=Fb_wanted  SaveFormat=Timeseries  SampleTime=-1
  Fb_wanted : Outport
  Ft_wanted : Outport  Port=2
  Fc_wanted : Outport  Port=3
  wires:
  Demux9/3 -> MATLAB Function6/3(M_z)
  Demux8/2 -> MATLAB Function6/1(F_y)
  Mux9/1 -> Fc_wanted/1, To Workspace6/1  "Fc_wanted"
  MATLAB Function/2(Ft2) -> Mux23/2  "Fb_wanted"
  Demux9/1 -> MATLAB Function6/2(M_x)
  MATLAB Function/3(Ft3) -> Mux23/3
  Demux9/2 -> MATLAB Function/1(My)
  MATLAB Function/8(Fb4) -> Mux24/4
  MATLAB Function6/1(F_c1) -> Mux9/1
  MATLAB Function/1(Ft1) -> Mux23/1  "Ft_wanted"
  Demux8/1 -> Terminator12/1
  Mux23/1 -> Ft_wanted/1, To Workspace7/1  "Ft_wanted"
  Mux24/1 -> Fb_wanted/1, To Workspace8/1  "Fb_wanted"
  MATLAB Function6/3(F_c3) -> Mux9/3
  MATLAB Function/5(Fb1) -> Mux24/1
  MATLAB Function/6(Fb2) -> Mux24/2
  MATLAB Function/7(Fb3) -> Mux24/3
  MATLAB Function/4(Ft4) -> Mux23/4
  Demux8/3 -> MATLAB Function/2(Fz)
  MATLAB Function6/2(F_c2) -> Mux9/2
  F_c_d/1 -> Demux8/1
  M_c_d/1 -> Demux9/1

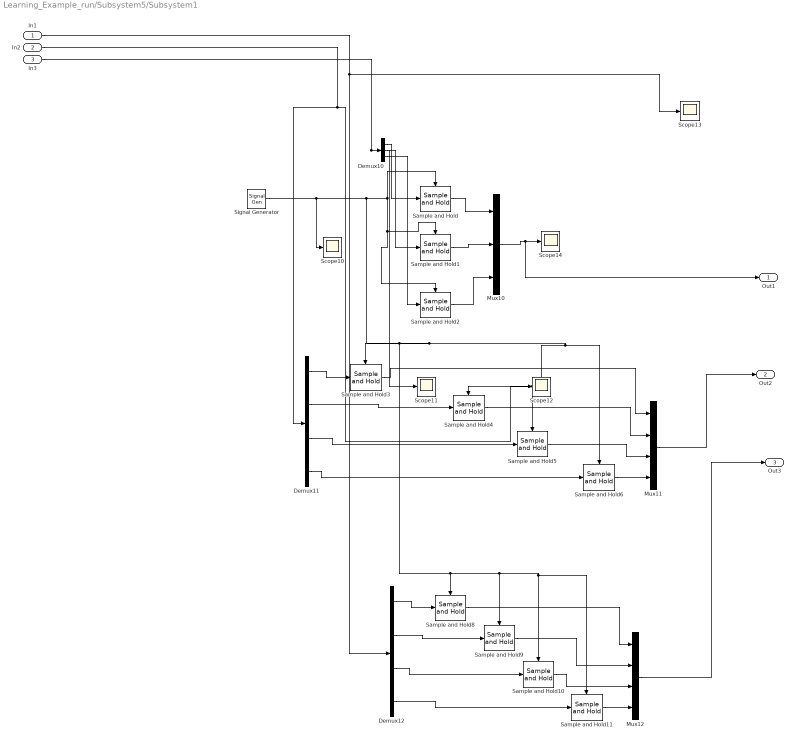
== system Learning_Example_run/Subsystem5/Subsystem1 ==
  In1 : Inport
  In2 : Inport  Port=2
  In3 : Inport  Port=3
  Demux10 : Demux  Outputs=3
  Demux11 : Demux
  Demux12 : Demux
  Mux10 : Mux  Inputs=3
  Mux11 : Mux
  Mux12 : Mux
  Sample and Hold{,1..6,8..11} (11 alike) : dspsigops/Sample and Hold  trig=Rising edge  initCond=0  latchinput=off
  Scope{10..14} (5 alike) : Scope
  Signal Generator : SignalGenerator  WaveForm=square  Frequency=fprop  Units=rad/sec
  Out1 : Outport
  Out2 : Outport  Port=2
  Out3 : Outport  Port=3
  wires:
  Demux12/1 -> Sample and Hold8/1
  Demux11/1 -> Sample and Hold3/1
  Signal Generator/1 -> Scope10/1, Sample and Hold11/Trigger, Sample and Hold10/Trigger, Sample and Hold9/Trigger, Sample and Hold8/Trigger, Sample and Hold4/Trigger, Sample and Hold5/Trigger, Sample and Hold6/Trigger, Sample and Hold3/Trigger, Sample and Hold/Trigger, Sample and Hold2/Trigger, Sample and Hold1/Trigger
  In2/1 -> Scope12/1, Demux11/1
  In3/1 -> Scope11/1, Demux10/1
  Demux10/3 -> Sample and Hold2/1
  Sample and Hold10/1 -> Mux12/3
  Sample and Hold/1 -> Mux10/1
  Demux12/4 -> Sample and Hold11/1
  Sample and Hold6/1 -> Mux11/4
  Demux10/1 -> Sample and Hold/1
  Mux10/1 -> Out1/1, Scope14/1
  Demux12/3 -> Sample and Hold10/1
  Sample and Hold8/1 -> Mux12/1
  Sample and Hold3/1 -> Mux11/1
  Sample and Hold5/1 -> Mux11/3
  Sample and Hold1/1 -> Mux10/2
  Sample and Hold11/1 -> Mux12/4
  In1/1 -> Scope13/1, Demux12/1
  Demux10/2 -> Sample and Hold1/1
  Demux11/2 -> Sample and Hold4/1
  Sample and Hold2/1 -> Mux10/3
  Sample and Hold4/1 -> Mux11/2
  Sample and Hold9/1 -> Mux12/2
  Demux11/3 -> Sample and Hold5/1
  Mux12/1 -> Out3/1
  Demux12/2 -> Sample and Hold9/1
  Demux11/4 -> Sample and Hold6/1
  Mux11/1 -> Out2/1

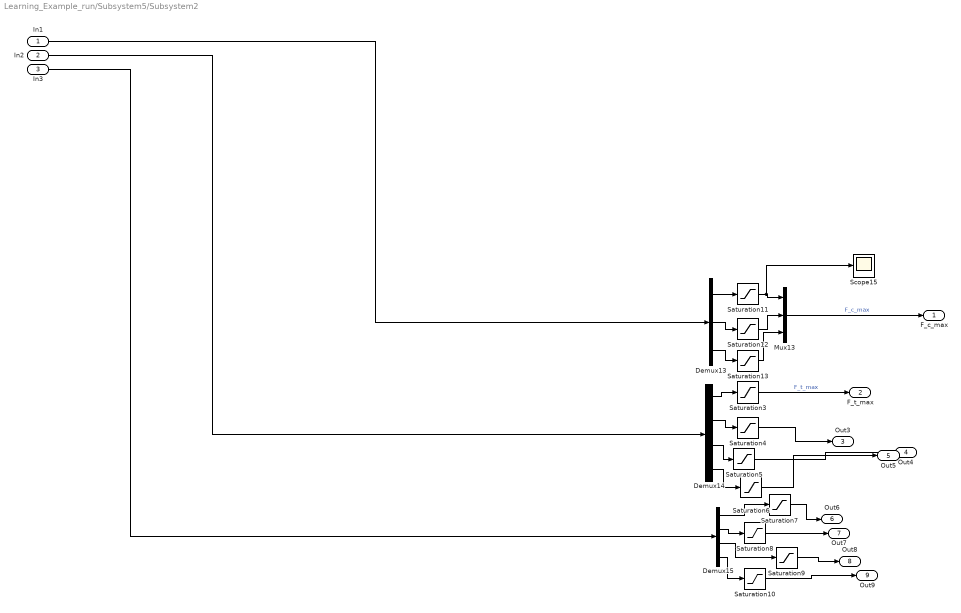
== system Learning_Example_run/Subsystem5/Subsystem2 ==
  In1 : Inport
  In2 : Inport  Port=2
  In3 : Inport  Port=3
  Demux13 : Demux  Outputs=3
  Demux14 : Demux
  Demux15 : Demux
  Mux13 : Mux  Inputs=3
  Saturation10 : Saturate  UpperLimit=Fb4_u  LowerLimit=Fb4_l
  Saturation11 : Saturate  UpperLimit=Fc1_u  LowerLimit=Fc1_l
  Saturation12 : Saturate  UpperLimit=Fc2_u  LowerLimit=Fc2_l
  Saturation13 : Saturate  UpperLimit=Fc3_u  LowerLimit=Fc3_l
  Saturation3 : Saturate  UpperLimit=Ft1_u  LowerLimit=Ft1_l
  Saturation4 : Saturate  UpperLimit=Ft2_u  LowerLimit=Ft2_l
  Saturation5 : Saturate  UpperLimit=Ft3_u  LowerLimit=Ft3_l
  Saturation6 : Saturate  UpperLimit=Ft4_u  LowerLimit=Ft4_l
  Saturation7 : Saturate  UpperLimit=Fb1_u  LowerLimit=Fb1_l
  Saturation8 : Saturate  UpperLimit=Fb2_u  LowerLimit=Fb2_l
  Saturation9 : Saturate  UpperLimit=Fb3_u  LowerLimit=Fb3_l
  Scope15 : Scope
  F_c_max : Outport
  F_t_max : Outport  Port=2
  Out3 : Outport  Port=3
  Out4 : Outport  Port=4
  Out5 : Outport  Port=5
  Out6 : Outport  Port=6
  Out7 : Outport  Port=7
  Out8 : Outport  Port=8
  Out9 : Outport  Port=9
  wires:
  Saturation11/1 -> Scope15/1, Mux13/1
  Demux13/2 -> Saturation12/1
  Saturation10/1 -> Out9/1
  Demux13/3 -> Saturation13/1
  Demux14/1 -> Saturation3/1
  Demux14/4 -> Saturation6/1
  In3/1 -> Demux15/1
  Demux14/3 -> Saturation5/1
  Demux13/1 -> Saturation11/1
  Saturation13/1 -> Mux13/3
  In1/1 -> Demux13/1
  Demux15/1 -> Saturation7/1
  Demux15/2 -> Saturation8/1
  Demux15/3 -> Saturation9/1
  Saturation12/1 -> Mux13/2
  Demux15/4 -> Saturation10/1
  Demux14/2 -> Saturation4/1
  Saturation9/1 -> Out8/1
  Saturation5/1 -> Out4/1
  In2/1 -> Demux14/1
  Saturation4/1 -> Out3/1
  Saturation7/1 -> Out6/1
  Mux13/1 -> F_c_max/1  "F_c_max"
  Saturation6/1 -> Out5/1
  Saturation3/1 -> F_t_max/1  "F_t_max"
  Saturation8/1 -> Out7/1

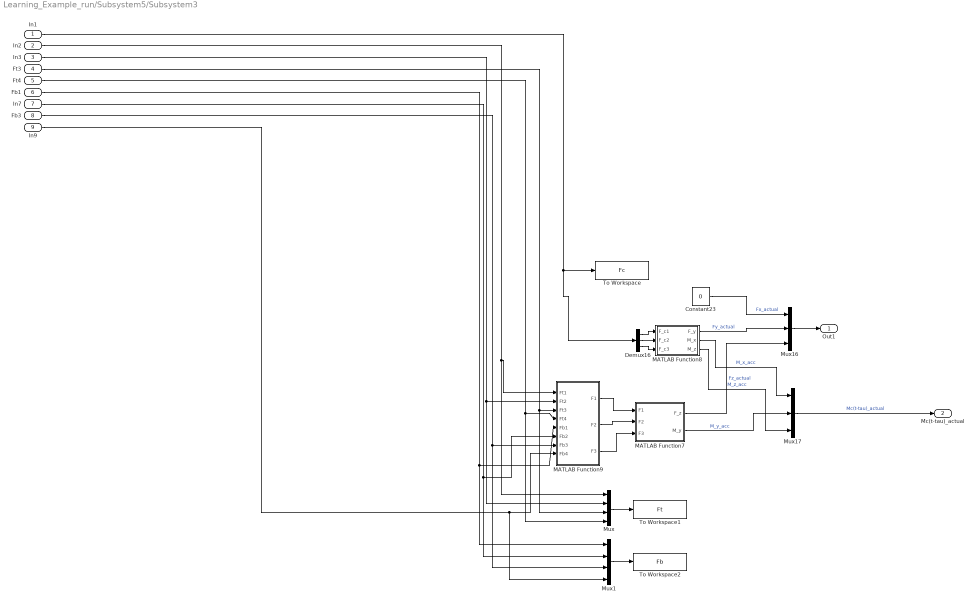
== system Learning_Example_run/Subsystem5/Subsystem3 ==
  In1 : Inport
  In2 : Inport  Port=2
  In3 : Inport  Port=3
  Ft3 : Inport  Port=4
  Ft4 : Inport  Port=5
  Fb1 : Inport  Port=6
  In7 : Inport  Port=7
  Fb3 : Inport  Port=8
  In9 : Inport  Port=9
  Constant23 : Constant  Value=0
  Demux16 : Demux  Outputs=3
  MATLAB Function7 : MATLAB Function  TreatAsAtomicUnit=on
  MATLAB Function8 : MATLAB Function  TreatAsAtomicUnit=on
  MATLAB Function9 : MATLAB Function  TreatAsAtomicUnit=on
  Mux : Mux
  Mux1 : Mux
  Mux16 : Mux  Inputs=3
  Mux17 : Mux  Inputs=3
  To Workspace : ToWorkspace  VariableName=Fc  SaveFormat=Timeseries  SampleTime=-1
  To Workspace1 : ToWorkspace  VariableName=Ft  SaveFormat=Timeseries  SampleTime=-1
  To Workspace2 : ToWorkspace  VariableName=Fb  SaveFormat=Timeseries  SampleTime=-1
  Out1 : Outport
  Mc(t-tau)_actual : Outport  Port=2
  wires:
  Demux16/2 -> MATLAB Function8/2(F_c2)
  In9/1 -> Mux1/4, MATLAB Function9/8(Fb4)
  In3/1 -> Mux/2, MATLAB Function9/2(Ft2)
  MATLAB Function7/1(F_z) -> Mux16/3  "Fz_actual"
  In1/1 -> Demux16/1, To Workspace/1
  Fb3/1 -> Mux1/3, MATLAB Function9/7(Fb3)
  MATLAB Function9/1(F1) -> MATLAB Function7/1(F1)
  Ft3/1 -> Mux/3, MATLAB Function9/3(Ft3)
  MATLAB Function8/1(F_y) -> Mux16/2  "Fy_actual"
  Fb1/1 -> Mux1/1, MATLAB Function9/5(Fb1)
  MATLAB Function8/3(M_z) -> Mux17/3  "M_z_acc"
  MATLAB Function7/2(M_y) -> Mux17/2  "M_y_acc"
  Mux17/1 -> Mc(t-tau)_actual/1  "Mc(t-tau)_actual"
  Ft4/1 -> Mux/4, MATLAB Function9/4(Ft4)
  MATLAB Function8/2(M_x) -> Mux17/1  "M_x_acc"
  In7/1 -> Mux1/2, MATLAB Function9/6(Fb2)
  MATLAB Function9/3(F3) -> MATLAB Function7/3(F3)
  Demux16/1 -> MATLAB Function8/1(F_c1)
  Constant23/1 -> Mux16/1  "Fx_actual"
  In2/1 -> Mux/1, MATLAB Function9/1(Ft1)
  MATLAB Function9/2(F2) -> MATLAB Function7/2(F2)
  Mux1/1 -> To Workspace2/1
  Demux16/3 -> MATLAB Function8/3(F_c3)
  Mux/1 -> To Workspace1/1
  Mux16/1 -> Out1/1

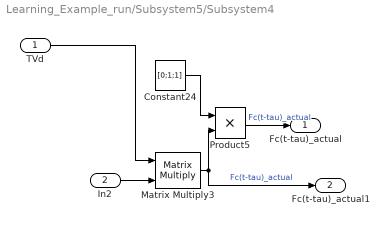
== system Learning_Example_run/Subsystem5/Subsystem4 ==
  TVd : Inport
  In2 : Inport  Port=2
  Constant24 : Constant  Value=[0;1;1]
  Matrix Multiply3 : Product  Multiplication=Matrix(*)
  Product5 : Product
  Fc(t-tau)_actual : Outport
  Fc(t-tau)_actual1 : Outport  Port=2
  wires:
  Matrix Multiply3/1 -> Fc(t-tau)_actual1/1, Product5/2  "Fc(t-tau)_actual"
  Constant24/1 -> Product5/1
  TVd/1 -> Matrix Multiply3/1
  Product5/1 -> Fc(t-tau)_actual/1  "Fc(t-tau)_actual"
  In2/1 -> Matrix Multiply3/2

== matlab function Learning_Example_run/Subsystem5/Subsystem/MATLAB Function ==
  data: My input; Ft1 output; Fz input; Ft2 output; Ft3 output; Ft4 output; Fb1 output; Fb2 output; Fb3 output; Fb4 output
function [Ft1, Ft2, Ft3, Ft4, Fb1, Fb2, Fb3, Fb4] = fixingpropulsionsmess(My, Fz)
xt_1 = 1.2598;
xb_1 = 2.2598;
xt_3 = -1.3402;
xb_3 = -1.3402;
x_t1 = xt_1;
x_b1 = xb_1;
x_t3 = xt_3;
x_b3 = xb_3;;

%alpha_1 = (-2*xt_1*(1/((xt_1/xb_1)-1))*(2 - (2*xb_3/xb_1)) - 4*xb_3)^2;
%alpha_2 = ((1/((xt_1/xb_1)-1))*(2-(2*xb_3/xb_1)))^2;
%alpha = alpha_1 + alpha_2;

%beta_1 = 2*My*((1/(2*xb_1))*(1 - (xt_1/xb_1)*(1/((xt_1/xb_1) -1))));
%beta_2 = 2*My*(1/((xt_1/xb_1) -1))*(1/(2*xb_1))*(1/((xt_1/xb_1) -1))*(2 - ((2*xb_3)/x_b1));
%beta_3 = 2*Fz*(1/(2*xb_1)*xt_1*(1/(xt_1/xb_1 -1)));
%beta_4 = 2*Fz*(-1/2*(1/(xt_1/xb_1 -1))*(1/(xt_1/xb_1 -1))*(2-2*xb_3/xb_1));
%beta = beta_1 + beta_2 + beta_3 + beta_4;

%a = beta/(2*alpha);
%y = 1/(2*xb_1)*(My - 2*xt_1*(1/(xt_1/xb_1 -1))*(-0.5*Fz + 2*(2 - 2*xb_3/xb_1)*a + 1/(2*xb_1)*My) - 4*xb_3*a);
%x = (1/(xt_1/xb_1 -1))*(-0.5*Fz + (2 - 2*xb_3/xb_1)*a + 1/(2*xb_1)*My);

a_num = 2/((2*xb_1 - 2*xt_1)^2) *(2*(4*xt_1 - 4*xb_3)*(My - Fz*0.5)) + 2*Fz + (4*My - Fz*(2 + 4*xt_1 - 4*xb_3))/(2*xb_1 - 2*xt_1);
a_den = -(2/((2*xb_1 - 2*xt_1)^2)*2*((4*xt_1 - 4*xb_3)^2) + 10 + (8*(4*xt_1 - 4*xb_3))/(-2*xt_1 + 2*xb_1));
a = a_num/a_den;

y = 1/(-2*xt_1 + 2*xb_1)*(a*(4*xt_1 - 4*xb_3) + My - 0.5*Fz);
x = -y - 2*a + Fz/2;
z = a;

Ft1 = x;
Ft2 = Ft1;
Ft3 = a;
Ft4 = Ft3;
Fb1 = y;
Fb2 = Fb1;
Fb3 = Ft3;
Fb4 = Ft3;
end

== matlab function Learning_Example_run/Subsystem1/MATLAB Function ==
  data: t input; u_0 output; u0 input; u1 input; u2 input; deltat input; u_1 output; u_2 output
function [u_0, u_1, u_2] = fcn(t, u0, u1, u2, deltat)

point = (t+deltat)/deltat;
point = round(point);
if point > length(u0)
    u_0 = u0(length(u0));
    u_1 = u1(length(u1));
    u_2 = u2(length(u2));
else
    u_0 = u0(point);
    u_1 = u1(point);
    u_2 = u2(point);
end

end

== matlab function Learning_Example_run/Subsystem5/Subsystem/MATLAB Function6 ==
  data: F_y input; F_c1 output; M_x input; M_z input; F_c2 output; F_c3 output
function [F_c1, F_c2, F_c3] = fcn(F_y, M_x, M_z)
%CATIA trans
TcgCatia = [1 0 0;
    0 -1 0;
    0 0 -1];

%Propeller arms - changed due to CATIA errors
c_1 = [-640.1998; 0; 506.566]*10^(-3);      %Control Back Top
c_2 = [-1040.1998; 0; -493.434]*10^(-3);    %Control Back Bottom
c_3 = [2259.8002; 0; -293.434]*10^(-3);     %Control Front

%Propeller arms - rotated
c_1 = TcgCatia*c_1;
c1 = transpose(c_1);
c_2 = TcgCatia*c_2;
c2 = transpose(c_2);
c_3 = TcgCatia*c_3;
c3 = transpose(c_3);

xc_1 = c1(1);
zc_1 = c1(3);

xc_2 = c2(1);
zc_2 = c2(3);

xc_3 = c3(1);
zc_3 = c3(3);

A_control = [1 1 1;
    zc_1 zc_2 zc_3;
    xc_1 xc_2 xc_3];
A_cinv = inv(A_control);
force_control = [F_y; M_x; M_z];
controlvec = A_cinv*force_control;
F_c1 = controlvec(1);
F_c2 = controlvec(2);
F_c3 = controlvec(3);
end

== matlab function Learning_Example_run/Subsystem5/Subsystem3/MATLAB Function7 ==
  data: F1 input; F_z output; F2 input; M_y output; F3 input
function [F_z, M_y] = fcn(F1, F2, F3)
xt_1 = 1.2598;
xb_1 = 2.2598;
xt_3 = -1.3402;
x_t1 = xt_1;
x_b1 = xb_1;
x_t3 = xt_3;

M_y = -100;
F_z = 0;

A_mat = [1 1;
    xt_1 xb_1];

A_inv = inv(A_mat);

force = [F1; F2];

back = A_mat*force;
backtrack = [4*F3; 4*F3*xt_3];
forceback = back+backtrack;
F_z = forceback(1);
M_y = forceback(2) + 0.15;
end

== matlab function Learning_Example_run/Subsystem5/Subsystem3/MATLAB Function8 ==
  data: F_c1 input; F_y output; M_x output; F_c2 input; F_c3 input; M_z output
function [F_y, M_x, M_z] = fcn(F_c1, F_c2, F_c3)

%CATIA trans
TcgCatia = [1 0 0;
    0 -1 0;
    0 0 -1];

%Propeller arms - changed due to CATIA errors
c_1 = [-640.1998; 0; 506.566]*10^(-3);      %Control Back Top
c_2 = [-1040.1998; 0; -493.434]*10^(-3);    %Control Back Bottom
c_3 = [2259.8002; 0; -293.434]*10^(-3);     %Control Front

%Propeller arms - rotated
c_1 = TcgCatia*c_1;
c1 = transpose(c_1);
c_2 = TcgCatia*c_2;
c2 = transpose(c_2);
c_3 = TcgCatia*c_3;
c3 = transpose(c_3);

xc_1 = c1(1);
zc_1 = c1(3);

xc_2 = c2(1);
zc_2 = c2(3);

xc_3 = c3(1);
zc_3 = c3(3);


Control_forces = [F_c1; F_c2; F_c3];

A_control = [1 1 1;
        zc_1 zc_2 zc_3;
        xc_1 xc_2 xc_3]; 
Control_vec_2 = A_control*Control_forces;
F_y = Control_vec_2(1);
M_x = Control_vec_2(2);
M_z = Control_vec_2(3);
end

== matlab function Learning_Example_run/Subsystem5/Subsystem3/MATLAB Function9 ==
  data: Ft1 input; F1 output; Ft2 input; F2 output; F3 output; Ft3 input; Ft4 input; Fb1 input; Fb2 input; Fb3 input; Fb4 input
function [F1, F2, F3] = fcn(Ft1, Ft2, Ft3, Ft4, Fb1, Fb2, Fb3, Fb4)
%F3 is one prop
%F1 is two props
%F2 is two props
F1 = 2*Ft1;
F2 = 2*Fb1;
F3 = Ft3;
end
